simulink model "environment_model"  (R2026a)
settings: Solver=VariableStepAuto
settings Model: Creator=GOD  LastModifiedBy=GOD

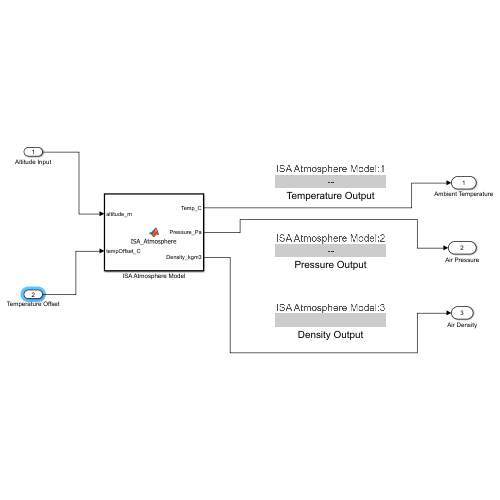
[thumbnail: Simulink's stored preview of the top-level diagram]
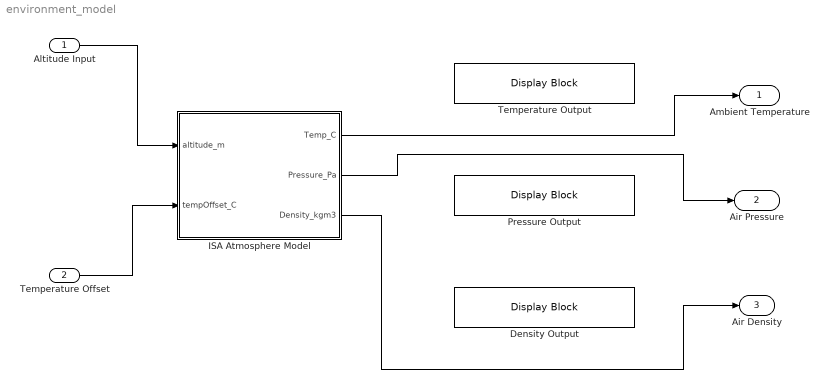
== system environment_model ==
  Altitude Input : Inport
  Temperature Offset : Inport  Port=2
  Density Output : DisplayBlock  Transparency=1  GridColor=[0.502, 0.502, 0.502]
  ISA Atmosphere Model : MATLAB Function  TreatAsAtomicUnit=on
  Pressure Output : DisplayBlock  Transparency=1  GridColor=[0.502, 0.502, 0.502]
  Temperature Output : DisplayBlock  Transparency=1  GridColor=[0.502, 0.502, 0.502]
  Ambient Temperature : Outport
  Air Pressure : Outport  Port=2
  Air Density : Outport  Port=3
  wires:
  Altitude Input/1 -> ISA Atmosphere Model/1(altitude_m)
  Temperature Offset/1 -> ISA Atmosphere Model/2(tempOffset_C)
  ISA Atmosphere Model/1(Temp_C) -> Ambient Temperature/1
  ISA Atmosphere Model/2(Pressure_Pa) -> Air Pressure/1
  ISA Atmosphere Model/3(Density_kgm3) -> Air Density/1

== matlab function environment_model/ISA Atmosphere Model ==
  data: altitude_m input; Temp_C output; tempOffset_C input; Pressure_Pa output; Density_kgm3 output
function [Temp_C, Pressure_Pa, Density_kgm3] = ISA_Atmosphere(altitude_m, tempOffset_C)
% International Standard Atmosphere (ISA) model
% Valid for troposphere (0-11 km) with a simple stratosphere extension
% These are universal physical constants (not Rotax-specific), so it
% is fine to keep them inside this function.

T0 = 288.15;      % Sea-level standard temperature, K (15 C)
P0 = 101325;      % Sea-level standard pressure, Pa
L  = 0.0065;      % Temperature lapse rate, K/m
R  = 287.05;      % Specific gas constant for air, J/(kg*K)
g0 = 9.80665;     % Standard gravity, m/s^2

if altitude_m <= 11000
    T_K = T0 - L*altitude_m;
    Pressure_Pa = P0 * (T_K/T0)^(g0/(L*R));
else
    T_11 = T0 - L*11000;
    P_11 = P0 * (T_11/T0)^(g0/(L*R));
    T_K = T_11;
    Pressure_Pa = P_11 * exp(-g0*(altitude_m-11000)/(R*T_11));
end

T_K = T_K + tempOffset_C;   % apply hot-day / cold-day deviation
Temp_C = T_K - 273.15;
Density_kgm3 = Pressure_Pa / (R*T_K);
end
